simulink model "GCI_Ctrl_PLL_C2000"  (R2024a)
settings: Solver=FixedStepDiscrete  StartTime=0.0  StopTime=8  FixedStep=Sim.ContSampleTime  RelTol=1e-3  EnableMultiTasking=on
values from neighbouring files (symbols this model uses):
  ADPTV = 1.3912    [ModelDD.sldd]
  Ctrl = 0    [ModelDD.sldd]
  EnableMonitors = 0    [ModelDD.sldd]
  FrcPwr = 1    [ModelDD.sldd]
  IdSp = 0.0    [ModelDD.sldd]
  IqSp = 0.0    [ModelDD.sldd]
  ModReq = 1    [ModelDD.sldd]
  PorISel = 0    [ModelDD.sldd]
  PSp = 0.0    [ModelDD.sldd]
  QSp = 0.0    [ModelDD.sldd]
  Sim : value not decoded    [ModelDD.sldd]
  Test = 0    [ModelDD.sldd]
  Var = 650.0    [ModelDD.sldd]
undefined symbols (not defined in the file or in its folder): DiscIntNeverNeededParam, Down, GPTRIP1SEL, GPTRIP2SEL, magnitude, P, TZ1, TZ2, Up
libraries: simulink x38, c2837xDlib x22, c2802xlib x15, slpidlib x9, spsMeanLib x9, spsCurrentMeasurementLib x7, spsThreePhaseVIMeasurementLib x5, spsVoltageMeasurementLib x5, spsTHDLib x4, spsSeriesRLCBranchLib x4, svdutilitieslib x3, c280xlib x3
(part 3 of 11)

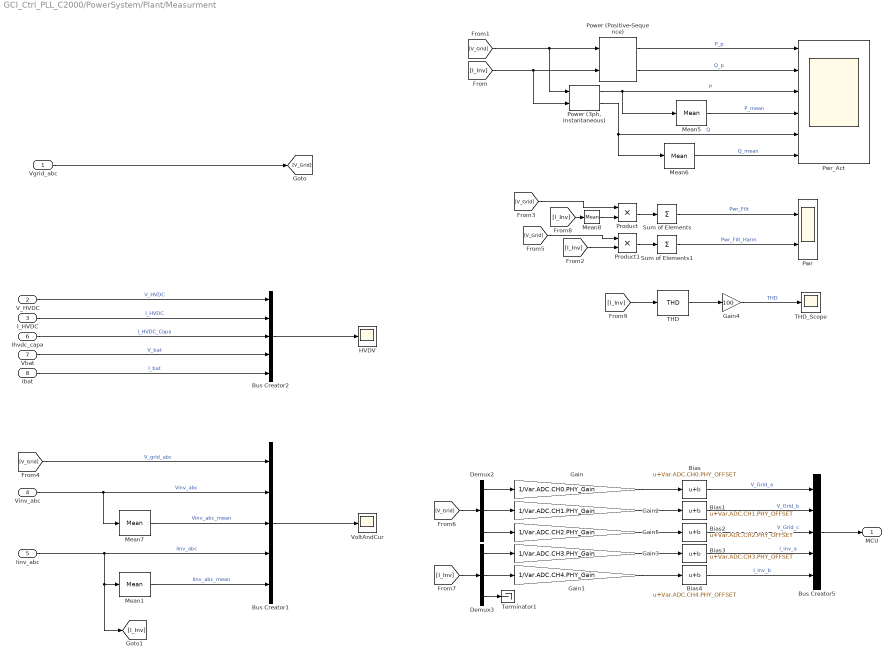
== system GCI_Ctrl_PLL_C2000/PowerSystem/Plant/Measurment ==
  Vgrid_abc : Inport
  V_HVDC : Inport  Port=2
  I_HVDC : Inport  Port=3
  Vinv_abc : Inport  Port=4
  Iinv_abc : Inport  Port=5
  Ihvdc_capa : Inport  Port=6
  Vbat : Inport  Port=7
  Ibat : Inport  Port=8
  Bias : Bias  Bias=Var.ADC.CH0.PHY_OFFSET  SaturateOnIntegerOverflow=off
  Bias1 : Bias  Bias=Var.ADC.CH1.PHY_OFFSET  SaturateOnIntegerOverflow=off
  Bias2 : Bias  Bias=Var.ADC.CH2.PHY_OFFSET  SaturateOnIntegerOverflow=off
  Bias3 : Bias  Bias=Var.ADC.CH3.PHY_OFFSET  SaturateOnIntegerOverflow=off
  Bias4 : Bias  Bias=Var.ADC.CH4.PHY_OFFSET  SaturateOnIntegerOverflow=off
  Bus Creator1 : BusCreator  Inputs=5
  Bus Creator2 : BusCreator  Inputs=5
  Bus Creator5 : BusCreator  Inputs=5
  Demux2 : Demux  Outputs=3
  Demux3 : Demux  Outputs=3
  Gain : Gain  Gain=1/Var.ADC.CH0.PHY_Gain
  Gain1 : Gain  Gain=1/Var.ADC.CH4.PHY_Gain
  Gain2 : Gain  Gain=1/Var.ADC.CH1.PHY_Gain
  Gain3 : Gain  Gain=1/Var.ADC.CH3.PHY_Gain
  Gain4 : Gain  Gain=100
  Gain5 : Gain  Gain=1/Var.ADC.CH2.PHY_Gain
  HVDV : Scope
  Mean1 : spsMeanLib/Mean  Freq=double(Var.PWM.Freq)  Vinit=0  Ts=0
  Mean5 : spsMeanLib/Mean  Freq=double(Var.Grid.Frq )  Vinit=0  Ts=0
  Mean6 : spsMeanLib/Mean  Freq=double(Var.Grid.Frq )  Vinit=0  Ts=0
  Mean7 : spsMeanLib/Mean  Freq=double(Var.PWM.Freq)  Vinit=0  Ts=0
  Mean8 : spsMeanLib/Mean  Freq="double(Var.PWM.Freq  )"  Vinit=0  Ts=0
  "Power (3ph, Instantaneous)" : spsPower3phInstantaneousLib/Power (3ph, Instantaneous)
  Power (Positive-Sequence) : spsPowerPositiveSequenceLib/Power (Positive-Sequence)  Freq=double(Var.Grid.Frq )  Vinit=[0, 0]  Iinit=[0, 0]  Ts=0
      settings: LibrarySourceBlock=|
      | sps_lib/Sensors and Measurements/Power
      | (Positive-Sequence)
  Product : Product
  Product1 : Product
  Pwr : Scope  NumInputPorts=2
  Pwr_Act : Scope  NumInputPorts=6
  Sum of Elements : Sum  Inputs=+
  Sum of Elements1 : Sum  Inputs=+
  THD : spsTHDLib/THD  Freq=double(Var.Grid.Frq )  Ts=0
  THD_Scope : Scope
  Terminator1 : Terminator
  VoltAndCur : Scope
  MCU : Outport  VectorParamsAs1DForOutWhenUnconnected=off
  wires:
  Iinv_abc/1 -> [I_Inv], Mean1/1, Bus Creator1/4  "Iinv_abc"
  Mean1/1 -> Bus Creator1/5  "Iinv_abc_mean"
  Mean7/1 -> Bus Creator1/3  "Vinv_abc_mean"
  Vinv_abc/1 -> Mean7/1, Bus Creator1/2  "Vinv_abc"
  Bus Creator2/1 -> HVDV/1
  Bus Creator1/1 -> VoltAndCur/1
  V_HVDC/1 -> Bus Creator2/1  "V_HVDC"
  I_HVDC/1 -> Bus Creator2/2  "I_HVDC"
  [V_Grid] -> Demux2/1
  [I_Inv] -> Demux3/1
  Demux2/1 -> Gain/1
  Demux3/2 -> Gain1/1
  Gain1/1 -> Bias4/1
  Gain3/1 -> Bias3/1
  Bias1/1 -> Bus Creator5/2  "V_Grid_b"
  Bias/1 -> Bus Creator5/1  "V_Grid_a"
  Bus Creator5/1 -> MCU/1
  Ihvdc_capa/1 -> Bus Creator2/3  "I_HVDC_Capa"
  Vbat/1 -> Bus Creator2/4  "V_bat"
  Ibat/1 -> Bus Creator2/5  "I_bat"
  Gain/1 -> Bias/1
  Demux2/2 -> Gain2/1
  Demux2/3 -> Gain5/1
  Gain2/1 -> Bias1/1
  Demux3/3 -> Terminator1/1
  Demux3/1 -> Gain3/1
  Power (Positive-Sequence)/1 -> Pwr_Act/1  "P_p"
  Power (Positive-Sequence)/2 -> Pwr_Act/2  "Q_p"
  Product/1 -> Sum of Elements/1
  THD/1 -> Gain4/1
  Gain4/1 -> THD_Scope/1  "THD"
  [I_Inv] -> "Power (3ph, Instantaneous)"/2, Power (Positive-Sequence)/2
  [V_Grid] -> "Power (3ph, Instantaneous)"/1, Power (Positive-Sequence)/1
  "Power (3ph, Instantaneous)"/1 -> Mean5/1, Pwr_Act/3  "P"
  "Power (3ph, Instantaneous)"/2 -> Pwr_Act/5, Mean6/1  "Q"
  Mean5/1 -> Pwr_Act/4  "P_mean"
  Mean6/1 -> Pwr_Act/6  "Q_mean"
  Mean8/1 -> Product/2
  Product1/1 -> Sum of Elements1/1
  Sum of Elements/1 -> Pwr/1  "Pwr_Filt"
  Sum of Elements1/1 -> Pwr/2  "Pwr_Filt_Harm"
  [I_Inv] -> Product1/2
  [V_Grid] -> Product/1
  [V_Grid] -> Product1/1
  [I_Inv] -> Mean8/1
  [I_Inv] -> THD/1
  [V_Grid] -> Bus Creator1/1  "V_grid_abc"
  Vgrid_abc/1 -> [V_Grid]
  Gain5/1 -> Bias2/1
  Bias2/1 -> Bus Creator5/3  "V_Grid_c"
  Bias3/1 -> Bus Creator5/4  "I_inv_a"
  Bias4/1 -> Bus Creator5/5  "I_inv_b"

== system GCI_Ctrl_PLL_C2000/PowerSystem/Plant/PWMGen1 ==
  Duty : Inport
  Constant : Constant  Value=0.5
  Deadtime : Subsystem  Commented=on
  Gain1 : Gain  Gain=2
  GreaterThan : RelationalOperator  Operator=>  RndMeth=Simplest  InputSameDT=off
  Mux : Mux  Inputs=2
  NOT : Logic  Operator=NOT  IconShape=distinctive  AllPortsSameDT=off  OutDataTypeStr=boolean
  Repeating Sequence : simulink/Sources/Repeating Sequence  rep_seq_t=[0 0.5/5000 1/5000]  rep_seq_y=[0 100 0]
  Scope : Scope  NumInputPorts=3
  Selector : Selector  InputPortWidth=6  IndexOptions=Index vector (dialog)  Indices=[1 4 2 5 3 6]  OutputSizes=1
  Subtract : Sum  Inputs=+-
  PWM : Outport  VectorParamsAs1DForOutWhenUnconnected=off
  wires:
  Mux/1 -> Selector/1
  Selector/1 -> Subtract/1
  Duty/1 -> GreaterThan/1, Scope/1
  Subtract/1 -> Gain1/1
  NOT/1 -> Mux/2
  Constant/1 -> Subtract/2
  Repeating Sequence/1 -> GreaterThan/2, Scope/2
  Gain1/1 -> PWM/1, Scope/3
  GreaterThan/1 -> Mux/1, NOT/1

== system GCI_Ctrl_PLL_C2000/PowerSystem/Plant/PWMGen2 ==
  Duty : Inport
  Constant : Constant  Value=0.5
  Deadtime : Subsystem  Commented=on
  Gain1 : Gain  Gain=2
  GreaterThan : RelationalOperator  Operator=>  RndMeth=Simplest  InputSameDT=off
  GreaterThan1 : RelationalOperator  Operator=>  RndMeth=Simplest  InputSameDT=off
  Mux : Mux  Inputs=2
  Repeating Sequence : simulink/Sources/Repeating Sequence  rep_seq_t=[0 0.5/5000 1/5000]  rep_seq_y=[0 100 0]
  Scope : Scope  NumInputPorts=4
  Selector : Selector  InputPortWidth=6  IndexOptions=Index vector (dialog)  Indices=[1 4 2 5 3 6]  OutputSizes=1
  Selector1 : Selector  InputPortWidth=6  IndexOptions=Index vector (dialog)  Indices=[1 2 3]  OutputSizes=1
  Selector2 : Selector  InputPortWidth=6  IndexOptions=Index vector (dialog)  Indices=[4 5 6]  OutputSizes=1
  Subtract : Sum  Inputs=+-
  PWM : Outport  VectorParamsAs1DForOutWhenUnconnected=off
  wires:
  Mux/1 -> Selector/1
  Gain1/1 -> Scope/4, PWM/1
  Repeating Sequence/1 -> GreaterThan1/1, Scope/3, GreaterThan/2
  Constant/1 -> Subtract/2
  Subtract/1 -> Gain1/1
  Duty/1 -> Scope/1, Selector2/1, Selector1/1
  Selector1/1 -> Scope/2, GreaterThan/1
  Selector2/1 -> GreaterThan1/2
  GreaterThan/1 -> Mux/1
  GreaterThan1/1 -> Mux/2
  Selector/1 -> Subtract/1

== system GCI_Ctrl_PLL_C2000/C2000_SW/Control/CommunicationMode/Serial Receive ==
  SCI_Rx_INT : TriggerPort  TriggerType=function-call  VariantControl=Variant
  Byte Pack1 : svdutilitieslib/Byte Pack  maskPackedDataType=uint8  datatypes={'single'}  byteAlign=1  blockPlatform=tic2000
      settings: LibrarySourceBlock=c2000lib/Target Communication/Byte Pack
  Byte Pack2 : svdutilitieslib/Byte Pack  maskPackedDataType=uint8  datatypes={'uint16'}  byteAlign=1  blockPlatform=tic2000
      settings: LibrarySourceBlock=c2000lib/Target Communication/Byte Pack
  Byte Unpack1 : svdutilitieslib/Byte Unpack  dimensions={[4]}  datatypes={'single'}  byteAlign=4  blockPlatform=tic2000
      settings: LibrarySourceBlock=c2000lib/Target Communication/Byte Unpack
  Data Store Read : DataStoreRead  Commented=on  DataStoreName=QSp  IndexOptions=Index vector (dialog)  Indices=1  OutputSizes=1
  Data Store Read1 : DataStoreRead  Commented=on  DataStoreName=PSp  IndexOptions=Index vector (dialog)  Indices=1  OutputSizes=1
  Data Store Read10 : DataStoreRead  DataStoreName=Irms  IndexOptions=Index vector (dialog)  Indices=1  OutputSizes=1
  Data Store Read11 : DataStoreRead  DataStoreName=Vdc  IndexOptions=Index vector (dialog)  Indices=1  OutputSizes=1
  Data Store Read12 : DataStoreRead  DataStoreName=Vrms  IndexOptions=Index vector (dialog)  Indices=1  OutputSizes=1
  Data Store Read13 : DataStoreRead  DataStoreName=w  IndexOptions=Index vector (dialog)  Indices=1  OutputSizes=1
  Data Store Read14 : DataStoreRead  DataStoreName=FailSw  IndexOptions=Index vector (dialog)  Indices=1  OutputSizes=1
  Data Store Read15 : DataStoreRead  DataStoreName=FailHw  IndexOptions=Index vector (dialog)  Indices=1  OutputSizes=1
  Data Store Read16 : DataStoreRead  DataStoreName=Fail  IndexOptions=Index vector (dialog)  Indices=1  OutputSizes=1
  Data Store Read17 : DataStoreRead  DataStoreName=SafeSt  IndexOptions=Index vector (dialog)  Indices=1  OutputSizes=1
  Data Store Read18 : DataStoreRead  DataStoreName=CtrlEn  IndexOptions=Index vector (dialog)  Indices=1  OutputSizes=1
  Data Store Read19 : DataStoreRead  DataStoreName=PllEnFb  IndexOptions=Index vector (dialog)  Indices=1  OutputSizes=1
  Data Store Read2 : DataStoreRead  Commented=on  DataStoreName=IqSp  IndexOptions=Index vector (dialog)  Indices=1  OutputSizes=1
  Data Store Read20 : DataStoreRead  DataStoreName=Synch  IndexOptions=Index vector (dialog)  Indices=1  OutputSizes=1
  Data Store Read21 : DataStoreRead  DataStoreName=Mode  IndexOptions=Index vector (dialog)  Indices=1  OutputSizes=1
  Data Store Read3 : DataStoreRead  Commented=on  DataStoreName=IdSp  IndexOptions=Index vector (dialog)  Indices=1  OutputSizes=1
  Data Store Read4 : DataStoreRead  Commented=on  DataStoreName=FrcPwr  IndexOptions=Index vector (dialog)  Indices=1  OutputSizes=1
  Data Store Read5 : DataStoreRead  Commented=on  DataStoreName=TestTrig  IndexOptions=Index vector (dialog)  Indices=1  OutputSizes=1
  Data Store Read6 : DataStoreRead  Commented=on  DataStoreName=EnaMon  IndexOptions=Index vector (dialog)  Indices=1  OutputSizes=1
  Data Store Read7 : DataStoreRead  Commented=on  DataStoreName=EnaPLL  IndexOptions=Index vector (dialog)  Indices=1  OutputSizes=1
  Data Store Read8 : DataStoreRead  Commented=on  DataStoreName=Sel_P_I  IndexOptions=Index vector (dialog)  Indices=1  OutputSizes=1
  Data Store Read9 : DataStoreRead  Commented=on  DataStoreName=ModReq  IndexOptions=Index vector (dialog)  Indices=1  OutputSizes=1
  Data Store Write : DataStoreWrite  DataStoreName=FrcPwr  IndexOptions=Index vector (dialog)  Indices=1  OutputSizes=1
  Data Store Write1 : DataStoreWrite  DataStoreName=TestTrig  IndexOptions=Index vector (dialog)  Indices=1  OutputSizes=1
  Data Store Write12 : DataStoreWrite  DataStoreName=IdSp  IndexOptions=Index vector (dialog)  Indices=1  OutputSizes=1
  Data Store Write13 : DataStoreWrite  DataStoreName=IqSp  IndexOptions=Index vector (dialog)  Indices=1  OutputSizes=1
  Data Store Write14 : DataStoreWrite  DataStoreName=PSp  IndexOptions=Index vector (dialog)  Indices=1  OutputSizes=1
  Data Store Write15 : DataStoreWrite  DataStoreName=QSp  IndexOptions=Index vector (dialog)  Indices=1  OutputSizes=1
  Data Store Write2 : DataStoreWrite  DataStoreName=EnaPLL  IndexOptions=Index vector (dialog)  Indices=1  OutputSizes=1
  Data Store Write3 : DataStoreWrite  DataStoreName=EnaMon  IndexOptions=Index vector (dialog)  Indices=1  OutputSizes=1
  Data Store Write4 : DataStoreWrite  DataStoreName=ModReq  IndexOptions=Index vector (dialog)  Indices=1  OutputSizes=1
  Data Store Write5 : DataStoreWrite  DataStoreName=Sel_P_I  IndexOptions=Index vector (dialog)  Indices=1  OutputSizes=1
  Data Type Conversion : DataTypeConversion  Commented=on  OutDataTypeStr=uint8  SaturateOnIntegerOverflow=off  RndMeth=Floor
  Demux : Demux
  Gain : Gain  Gain=single(2.^(0:4))  ParamDataTypeStr=single
  Mux : Mux  Commented=on
  Mux1 : Mux  Commented=on  Inputs=6
  Mux2 : Mux  Inputs=2
  Mux3 : Mux
  Mux4 : Mux  Inputs=5
  Mux5 : Mux
  SCI Receive : c280xlib/SCI Receive  sciModule=A  dataHead='SS'  headerCheckMaxCount=16  dataTail='EE'  dataType=uint8  dataLenOptions=Length via dialog  dataDim=17  maxDataLength=1  initValue=0  errOption=Output the last received value  errValue=0  sampleTime=-1  blockingMode=on  timeOut=1  outputStatus=off
  SCI Transmit : c280xlib/SCI Transmit  sciModule=A  dataHead='SS'  dataTail='EE'  frameSize=1  blockingMode=on  outputStatus=off
  Selector : Selector  InputPortWidth=17  IndexOptions=Index vector (dialog)  Indices=1:16  OutputSizes=1
  Selector1 : Selector  InputPortWidth=17  IndexOptions=Index vector (dialog)  Indices=17  OutputSizes=1
  Sum of Elements : Sum  Inputs=+  OutDataTypeStr=uint8
  unParse : Subsystem
  wires:
  Selector1/1 -> unParse/1(Data)
  unParse/1(ForcePwr) -> Data Store Write/1
  unParse/5(P_or_I) -> Data Store Write5/1
  unParse/2(TestTrigger) -> Data Store Write1/1
  unParse/3(EnaMon) -> Data Store Write3/1
  unParse/4(EnaPLL) -> Data Store Write2/1
  SCI Receive/1 -> Selector1/1, Selector/1
  Byte Unpack1/1 -> Demux/1
  Demux/2 -> Data Store Write13/1
  Demux/1 -> Data Store Write12/1
  Demux/3 -> Data Store Write14/1
  Demux/4 -> Data Store Write15/1
  Data Store Read/1 -> Mux/4
  Data Store Read1/1 -> Mux/3
  Data Store Read2/1 -> Mux/2
  Data Store Read3/1 -> Mux/1
  Mux3/1 -> Byte Pack1/1
  Selector/1 -> Byte Unpack1/1
  Data Store Read4/1 -> Mux1/1
  Data Store Read5/1 -> Mux1/2
  Data Store Read6/1 -> Mux1/3
  Data Store Read7/1 -> Mux1/4
  Data Store Read8/1 -> Mux1/5
  Mux1/1 -> Data Type Conversion/1
  Mux5/1 -> Mux2/2
  unParse/6(Mod) -> Data Store Write4/1
  Data Store Read9/1 -> Mux1/6
  Byte Pack1/1 -> Mux2/1  "Transmitted signal"
  Mux2/1 -> SCI Transmit/1
  Data Store Read10/1 -> Mux3/1
  Data Store Read11/1 -> Mux3/2
  Data Store Read12/1 -> Mux3/3
  Data Store Read13/1 -> Mux3/4
  Gain/1 -> Sum of Elements/1
  Data Store Read16/1 -> Mux4/1
  Data Store Read17/1 -> Mux4/2
  Data Store Read20/1 -> Mux4/3
  Data Store Read18/1 -> Mux4/4
  Data Store Read19/1 -> Mux4/5
  Mux4/1 -> Gain/1
  Data Store Read14/1 -> Byte Pack2/1
  Data Store Read21/1 -> Mux5/1
  Sum of Elements/1 -> Mux5/4
  Data Store Read15/1 -> Mux5/3
  Byte Pack2/1 -> Mux5/2  "Transmitted signal"

== system GCI_Ctrl_PLL_C2000/C2000_SW/CtrlLoop/ADC Scaling/ADC Scaling 3 Cur ==
  note: Data Collection
  note: Data Collection
  Ch1 : Inport
  Ch2 : Inport  Port=2
  Ch3 : Inport  Port=3
  Ch4 : Inport  Port=4
  Ch5 : Inport  Port=5
  Ch6 : Inport  Port=6
  SPO : Inport  Port=7
  PllEn : Inport  Port=8
  Add5 : Sum  Inputs=--  OutDataTypeStr=single
  Bus Creator : BusCreator  Commented=on  Inputs=6
  Bus Creator1 : BusCreator  Inputs=8
  Bus Selector : BusSelector  OutputSignals=VaActMeas
  Bus Selector1 : BusSelector  OutputSignals=VbActMeas
  Bus Selector2 : BusSelector  OutputSignals=IaActMeas
  Bus Selector3 : BusSelector  OutputSignals=IbActMeas
  Bus Selector4 : BusSelector  OutputSignals=IcActMeas
  Bus Selector5 : BusSelector  OutputSignals=VdcActMeas
  From : From  Commented=on  GotoTag=VaMeas
  From1 : From  Commented=on  GotoTag=VbMeas
  From2 : From  Commented=on  GotoTag=VcMeas
  From3 : From  Commented=on  GotoTag=IaMeas
  From4 : From  Commented=on  GotoTag=IbMeas
  From5 : From  Commented=on  GotoTag=VdcMeas
  Mux : Mux  Inputs=3
  Mux1 : Mux  Inputs=3
  NOT : Logic  Commented=on  Operator=NOT  IconShape=distinctive  AllPortsSameDT=off  OutDataTypeStr=boolean
  RemoveDCOffset : Subsystem  Variant=on  VariantControl=Variant1
      settings: PortSchema="{\"entries\":[{\"content\":{\"sides\":[{\"content\":{\"connectorIds\":[\"In1\"]},\"type\":\"ConnectorPlacement.EquallySpacedRectSide\",\"uuid\":\"cc4d9f7f-47aa-49df-af9b-f6b1a27a89d1\"},{\"content\":{\"connectorIds\":[\"Out1\",\"Out2\"],\"side\":\"RIGHT\"},\"type\":\"ConnectorPlacement.EquallySpacedRectSide\",\"uuid\":\"3802b5cc-b213-4712-8426-72153f4334cb\"},{\"content\":{\"connectorIds\":[\"In2\"],\"side\":\"TOP\"},\"type\":\"ConnectorPlacement.EquallySpacedRectSide\",\"uuid\":\"ab2b61dd-4b54-4d07-8aa7-d75851ccd714\"}]},\"type\":\"ConnectorPlacement.EquallySpacedConnector\",\"uuid\":\"275358d2-d3f0-4fc6-bdde-8d29d39068fc\"}],\"packageUris\":[\"http://schema.mathworks.com/mf0/Connector/R2020b\"],\"version\":\"1.0\"}"
  Scaling : Subsystem  mask{ADC_Gain=Var.ADC_CH0_Gain, ADC_Off=Var.ADC_CH0_OFFSET, Res=Var.ADC_Res, ADC_Gain_Phy=Var.ADC_CH0_PHY_Gain, ADC_Off_Phy=Var.ADC_CH0_PHY_OFFSET}
      mask prompts: ADC_Gain "ADC Gain"; ADC_Off "ADC Offset"; Res "Resoloution"; ADC_Gain_Phy "Physical Gain"; ADC_Off_Phy "Physical Offset"
  Scaling1 : Subsystem  mask{ADC_Gain=Var.ADC_CH1_Gain, ADC_Off=Var.ADC_CH1_OFFSET, Res=Var.ADC_Res, ADC_Gain_Phy=Var.ADC_CH1_PHY_Gain, ADC_Off_Phy=Var.ADC_CH1_PHY_OFFSET}
      mask prompts: ADC_Gain "ADC Gain"; ADC_Off "ADC Offset"; Res "Resoloution"; ADC_Gain_Phy "Physical Gain"; ADC_Off_Phy "Physical Offset"
  Scaling2 : Subsystem  mask{ADC_Gain=Var.ADC_CH2_Gain, ADC_Off=Var.ADC_CH2_OFFSET, Res=Var.ADC_Res, ADC_Gain_Phy=Var.ADC_CH2_PHY_Gain, ADC_Off_Phy=Var.ADC_CH2_PHY_OFFSET}
      mask prompts: ADC_Gain "ADC Gain"; ADC_Off "ADC Offset"; Res "Resoloution"; ADC_Gain_Phy "Physical Gain"; ADC_Off_Phy "Physical Offset"
  Scaling3 : Subsystem  mask{ADC_Gain=Var.ADC_CH3_Gain, ADC_Off=Var.ADC_CH3_OFFSET, Res=Var.ADC_Res, ADC_Gain_Phy=Var.ADC_CH3_PHY_Gain, ADC_Off_Phy=Var.ADC_CH3_PHY_OFFSET}
      mask prompts: ADC_Gain "ADC Gain"; ADC_Off "ADC Offset"; Res "Resoloution"; ADC_Gain_Phy "Physical Gain"; ADC_Off_Phy "Physical Offset"
  Scaling4 : Subsystem  mask{ADC_Gain=Var.ADC_CH4_Gain, ADC_Off=Var.ADC_CH4_OFFSET, Res=Var.ADC_Res, ADC_Gain_Phy=Var.ADC_CH4_PHY_Gain, ADC_Off_Phy=Var.ADC_CH4_PHY_OFFSET}
      mask prompts: ADC_Gain "ADC Gain"; ADC_Off "ADC Offset"; Res "Resoloution"; ADC_Gain_Phy "Physical Gain"; ADC_Off_Phy "Physical Offset"
  Scaling5 : Subsystem  mask{ADC_Gain=Var.ADC_CH5_Gain, ADC_Off=Var.ADC_CH5_OFFSET, Res=Var.ADC_Res, ADC_Gain_Phy=Var.ADC_CH5_PHY_Gain, ADC_Off_Phy=Var.ADC_CH5_PHY_OFFSET}
      mask prompts: ADC_Gain "ADC Gain"; ADC_Off "ADC Offset"; Res "Resoloution"; ADC_Gain_Phy "Physical Gain"; ADC_Off_Phy "Physical Offset"
  Subsystem : Subsystem
  Sum : Sum  Inputs=|+-
  Terminator : Terminator
  Unit Delay : UnitDelay  Commented=on  SampleTime=-1  HasFrameUpgradeWarning=on
  Vgrid_abc : Outport  OutDataTypeStr=single  VectorParamsAs1DForOutWhenUnconnected=off
  I_abc : Outport  Port=2  OutDataTypeStr=single  VectorParamsAs1DForOutWhenUnconnected=off
  Vhvdc : Outport  Port=3  OutDataTypeStr=single  VectorParamsAs1DForOutWhenUnconnected=off
  Mon : Outport  Port=4  OutDataTypeStr=single  VectorParamsAs1DForOutWhenUnconnected=off
  wires:
  RemoveDCOffset/2(VabcGridOff) -> Terminator/1
  NOT/1 -> Unit Delay/1
  Unit Delay/1 -> NOT/1
  SPO/1 -> Subsystem/Enable
  Subsystem/1(Offset) -> Sum/2
  Sum/1 -> I_abc/1, Bus Creator1/8  "Iabc_NoDcOff"
  RemoveDCOffset/1(VabcGridAdj) -> Bus Creator1/7, Vgrid_abc/1  "Vabc_NoDcOff"
  Bus Selector5/1 -> Bus Creator1/6  "<VdcActMeas>"
  Bus Selector4/1 -> Bus Creator1/5  "<IcActMeas>"
  Bus Selector3/1 -> Bus Creator1/4  "<IbActMeas>"
  Bus Selector2/1 -> Bus Creator1/3  "<IaActMeas>"
  Bus Selector1/1 -> Bus Creator1/2  "<VbActMeas>"
  Bus Selector/1 -> Bus Creator1/1  "<VaActMeas>"
  [VbMeas] -> Bus Selector1/1
  [VaMeas] -> Bus Selector/1
  [IaMeas] -> Bus Selector2/1
  [IcMeas] -> Bus Selector4/1
  [VdcMeas] -> Bus Selector5/1
  [IbMeas] -> Bus Selector3/1
  Ch4/1 -> Scaling3/1(CH)
  From5/1 -> Bus Creator/6
  Scaling5/2(CH_Meas) -> Vhvdc/1
  Scaling5/1(Meas) -> [VdcMeas]
  Ch6/1 -> Scaling5/1(CH)
  From3/1 -> Bus Creator/4
  From2/1 -> Bus Creator/3
  From4/1 -> Bus Creator/5
  From/1 -> Bus Creator/1
  Scaling4/2(CH_Meas) -> Mux1/3
  Scaling1/2(CH_Meas) -> Mux/2, Add5/2
  Scaling2/1(Mon) -> [IaMeas]
  Scaling3/2(CH_Meas) -> Mux1/2
  Ch5/1 -> Scaling4/1(CH)
  Scaling4/1(Meas) -> [IcMeas]
  Scaling3/1(Meas) -> [IbMeas]
  Scaling1/1(Mon) -> [VbMeas]
  Scaling/2(CH_Meas) -> Add5/1, Mux/1
  Scaling/1(Mon) -> [VaMeas]
  Scaling2/2(CH_Meas) -> Mux1/1
  Mux1/1 -> Sum/1, Subsystem/1(IabcActMeas)  "IabcActMeas"
  Mux/1 -> RemoveDCOffset/1(VabcGrid)  "VgabcActMeas"
  Ch1/1 -> Scaling/1(CH)
  Ch3/1 -> Scaling2/1(CH)
  Ch2/1 -> Scaling1/1(CH)
  From1/1 -> Bus Creator/2
  Bus Creator1/1 -> Mon/1  "ScaleMon"
  Add5/1 -> Mux/3  "Vc"
  PllEn/1 -> [A1]
  [A1] -> RemoveDCOffset/2(Rst)

== system GCI_Ctrl_PLL_C2000/C2000_SW/CtrlLoop/ADC Scaling/ADC Scaling 3 Volts ==
  note: Data Collection
  note: Data Collection
  Ch1 : Inport
  Ch2 : Inport  Port=2
  Ch3 : Inport  Port=3
  Ch4 : Inport  Port=4
  Ch5 : Inport  Port=5
  Ch6 : Inport  Port=6
  SPO : Inport  Port=7
  Add5 : Sum  Inputs=--  OutDataTypeStr=single
  Bus Creator : BusCreator  Commented=on  Inputs=6
  Bus Creator1 : BusCreator  Inputs=8
  Bus Selector : BusSelector  OutputSignals=VaActMeas
  Bus Selector1 : BusSelector  OutputSignals=VbActMeas
  Bus Selector2 : BusSelector  OutputSignals=VcActMeas
  Bus Selector3 : BusSelector  OutputSignals=IaActMeas
  Bus Selector4 : BusSelector  OutputSignals=IbActMeas
  Bus Selector5 : BusSelector  OutputSignals=VdcActMeas
  From : From  Commented=on  GotoTag=VaMeas
  From1 : From  Commented=on  GotoTag=VbMeas
  From2 : From  Commented=on  GotoTag=VcMeas
  From3 : From  Commented=on  GotoTag=IaMeas
  From4 : From  Commented=on  GotoTag=IbMeas
  From5 : From  Commented=on  GotoTag=VdcMeas
  Mux : Mux  Inputs=3
  Mux1 : Mux  Inputs=3
  NOT : Logic  Commented=on  Operator=NOT  IconShape=distinctive  AllPortsSameDT=off  OutDataTypeStr=boolean
  RemoveDCOffset : Subsystem  Variant=on  VariantControl=Variant1
  Scaling : Subsystem  mask{ADC_Gain=Var.ADC_CH0_Gain, ADC_Off=Var.ADC_CH0_OFFSET, Res=Var.ADC_Res, ADC_Gain_Phy=Var.ADC_CH0_PHY_Gain, ADC_Off_Phy=Var.ADC_CH0_PHY_OFFSET}
      mask prompts: ADC_Gain "ADC Gain"; ADC_Off "ADC Offset"; Res "Resoloution"; ADC_Gain_Phy "Physical Gain"; ADC_Off_Phy "Physical Offset"
  Scaling1 : Subsystem  mask{ADC_Gain=Var.ADC_CH1_Gain, ADC_Off=Var.ADC_CH1_OFFSET, Res=Var.ADC_Res, ADC_Gain_Phy=Var.ADC_CH1_PHY_Gain, ADC_Off_Phy=Var.ADC_CH1_PHY_OFFSET}
      mask prompts: ADC_Gain "ADC Gain"; ADC_Off "ADC Offset"; Res "Resoloution"; ADC_Gain_Phy "Physical Gain"; ADC_Off_Phy "Physical Offset"
  Scaling2 : Subsystem  mask{ADC_Gain=Var.ADC_CH2_Gain, ADC_Off=Var.ADC_CH2_OFFSET, Res=Var.ADC_Res, ADC_Gain_Phy=Var.ADC_CH2_PHY_Gain, ADC_Off_Phy=Var.ADC_CH2_PHY_OFFSET}
      mask prompts: ADC_Gain "ADC Gain"; ADC_Off "ADC Offset"; Res "Resoloution"; ADC_Gain_Phy "Physical Gain"; ADC_Off_Phy "Physical Offset"
  Scaling3 : Subsystem  mask{ADC_Gain=Var.ADC_CH3_Gain, ADC_Off=Var.ADC_CH3_OFFSET, Res=Var.ADC_Res, ADC_Gain_Phy=Var.ADC_CH3_PHY_Gain, ADC_Off_Phy=Var.ADC_CH3_PHY_OFFSET}
      mask prompts: ADC_Gain "ADC Gain"; ADC_Off "ADC Offset"; Res "Resoloution"; ADC_Gain_Phy "Physical Gain"; ADC_Off_Phy "Physical Offset"
  Scaling4 : Subsystem  mask{ADC_Gain=Var.ADC_CH4_Gain, ADC_Off=Var.ADC_CH4_OFFSET, Res=Var.ADC_Res, ADC_Gain_Phy=Var.ADC_CH4_PHY_Gain, ADC_Off_Phy=Var.ADC_CH4_PHY_OFFSET}
      mask prompts: ADC_Gain "ADC Gain"; ADC_Off "ADC Offset"; Res "Resoloution"; ADC_Gain_Phy "Physical Gain"; ADC_Off_Phy "Physical Offset"
  Scaling5 : Subsystem  mask{ADC_Gain=Var.ADC_CH5_Gain, ADC_Off=Var.ADC_CH5_OFFSET, Res=Var.ADC_Res, ADC_Gain_Phy=Var.ADC_CH5_PHY_Gain, ADC_Off_Phy=Var.ADC_CH5_PHY_OFFSET}
      mask prompts: ADC_Gain "ADC Gain"; ADC_Off "ADC Offset"; Res "Resoloution"; ADC_Gain_Phy "Physical Gain"; ADC_Off_Phy "Physical Offset"
  Subsystem : Subsystem
  Sum : Sum  Inputs=|+-
  Terminator : Terminator
  Unit Delay : UnitDelay  Commented=on  SampleTime=-1  HasFrameUpgradeWarning=on
  Vgrid_abc : Outport  OutDataTypeStr=single  VectorParamsAs1DForOutWhenUnconnected=off
  I_abc : Outport  Port=2  OutDataTypeStr=single  VectorParamsAs1DForOutWhenUnconnected=off
  Vhvdc : Outport  Port=3  OutDataTypeStr=single  VectorParamsAs1DForOutWhenUnconnected=off
  Mon : Outport  Port=4  OutDataTypeStr=single  VectorParamsAs1DForOutWhenUnconnected=off
  wires:
  Bus Creator1/1 -> Mon/1  "ScaleMon"
  From1/1 -> Bus Creator/2
  Ch2/1 -> Scaling1/1(CH)
  Ch3/1 -> Scaling2/1(CH)
  Ch1/1 -> Scaling/1(CH)
  Mux/1 -> RemoveDCOffset/1(VabcGrid)  "VgabcActMeas"
  Mux1/1 -> Subsystem/1(IabcActMeas), Sum/1  "IabcActMeas"
  Add5/1 -> Mux1/3  "Ic"
  Scaling2/2(CH_Meas) -> Mux/3
  Scaling/1(Mon) -> [VaMeas]
  Scaling/2(CH_Meas) -> Mux/1
  Scaling1/1(Mon) -> [VbMeas]
  Scaling3/1(Meas) -> [IaMeas]
  Scaling4/1(Meas) -> [IbMeas]
  Ch5/1 -> Scaling4/1(CH)
  Scaling3/2(CH_Meas) -> Add5/1, Mux1/1
  Scaling2/1(Mon) -> [VcMeas]
  Scaling1/2(CH_Meas) -> Mux/2
  Scaling4/2(CH_Meas) -> Add5/2, Mux1/2
  From/1 -> Bus Creator/1
  From4/1 -> Bus Creator/5
  From2/1 -> Bus Creator/3
  From3/1 -> Bus Creator/4
  Ch6/1 -> Scaling5/1(CH)
  Scaling5/1(Meas) -> [VdcMeas]
  Scaling5/2(CH_Meas) -> Vhvdc/1
  From5/1 -> Bus Creator/6
  Ch4/1 -> Scaling3/1(CH)
  [IbMeas] -> Bus Selector4/1
  [VdcMeas] -> Bus Selector5/1
  [VcMeas] -> Bus Selector2/1
  [IaMeas] -> Bus Selector3/1
  [VaMeas] -> Bus Selector/1
  [VbMeas] -> Bus Selector1/1
  Bus Selector/1 -> Bus Creator1/1  "<VaActMeas>"
  Bus Selector1/1 -> Bus Creator1/2  "<VbActMeas>"
  Bus Selector2/1 -> Bus Creator1/3  "<VcActMeas>"
  Bus Selector3/1 -> Bus Creator1/4  "<IaActMeas>"
  Bus Selector4/1 -> Bus Creator1/5  "<IbActMeas>"
  Bus Selector5/1 -> Bus Creator1/6  "<VdcActMeas>"
  RemoveDCOffset/1(VabcGridAdj) -> Vgrid_abc/1, Bus Creator1/7  "Vabc_NoDcOff"
  Sum/1 -> Bus Creator1/8, I_abc/1  "Iabc_NoDcOff"
  Subsystem/1(Offset) -> Sum/2
  SPO/1 -> Subsystem/Enable
  Unit Delay/1 -> NOT/1
  NOT/1 -> Unit Delay/1
  RemoveDCOffset/2(VabcGridOff) -> Terminator/1

== system GCI_Ctrl_PLL_C2000/C2000_SW/CtrlLoop/ADCs/HW ==
  note: Data Collection
  Meas : Inport
  ADC1 : c2802xlib/ADC  Commented=on  blkParamProc=C2000_Type4  ADCModule=C  samplingMode=Single sample mode  ADCResolution=12-bit (Single-ended input)  useSOC1=SOC0  useSOC2=SOC0_SOC1  SOCAcquisitionWindow=75  SOCTriggerSource=ePWM4_ADCSOCA  SOCInterruptTrigger=No ADCINT  Ts=-1  dType=uint16  postInterrupt=off  interruptSel=ADCINT2  ADCINTContinuous=off  endma=off  chdma=1  conv1=ADCINA0  conv2=ADCINA0 and ADCINB0  conv1_Type4=ADCIN2  conv2_Type4=ADCIN2 and ADCIN3
  ADC10 : c2802xlib/ADC  blkParamProc=C2000_Type4  ADCModule=C  samplingMode=Single sample mode  ADCResolution=12-bit (Single-ended input)  useSOC1=SOC0  useSOC2=SOC0_SOC1  SOCAcquisitionWindow=75  SOCTriggerSource=ePWM4_ADCSOCA  SOCInterruptTrigger=No ADCINT  Ts=-1  dType=uint32  postInterrupt=off  interruptSel=ADCINT2  ADCINTContinuous=off  endma=off  chdma=1  conv1=ADCINA0  conv2=ADCINA0 and ADCINB0  conv1_Type4=ADCIN2  conv2_Type4=ADCIN2 and ADCIN3
  ADC11 : c2802xlib/ADC  blkParamProc=C2000_Type4  ADCModule=A  samplingMode=Single sample mode  ADCResolution=12-bit (Single-ended input)  useSOC1=SOC1  useSOC2=SOC0_SOC1  SOCAcquisitionWindow=75  SOCTriggerSource=ePWM4_ADCSOCA  SOCInterruptTrigger=No ADCINT  Ts=-1  dType=uint32  postInterrupt=off  interruptSel=ADCINT1  ADCINTContinuous=off  endma=off  chdma=1  conv1=ADCINA0  conv2=ADCINA0 and ADCINB0  conv1_Type4=ADCIN1  conv2_Type4=ADCIN4 and ADCIN5
  ADC12 : c2802xlib/ADC  blkParamProc=C2000_Type4  ADCModule=A  samplingMode=Single sample mode  ADCResolution=12-bit (Single-ended input)  useSOC1=SOC2  useSOC2=SOC0_SOC1  SOCAcquisitionWindow=75  SOCTriggerSource=ePWM4_ADCSOCA  SOCInterruptTrigger=No ADCINT  Ts=-1  dType=uint32  postInterrupt=off  interruptSel=ADCINT4  ADCINTContinuous=off  endma=off  chdma=1  conv1=ADCINA0  conv2=ADCINA0 and ADCINB0  conv1_Type4=ADCIN2  conv2_Type4=ADCIN4 and ADCIN5
  ADC2 : c2802xlib/ADC  Commented=on  blkParamProc=C2000_Type4  ADCModule=C  samplingMode=Single sample mode  ADCResolution=12-bit (Single-ended input)  useSOC1=SOC1  useSOC2=SOC0_SOC1  SOCAcquisitionWindow=75  SOCTriggerSource=ePWM4_ADCSOCA  SOCInterruptTrigger=No ADCINT  Ts=-1  dType=uint16  postInterrupt=off  interruptSel=ADCINT4  ADCINTContinuous=off  endma=off  chdma=1  conv1=ADCINA0  conv2=ADCINA0 and ADCINB0  conv1_Type4=ADCIN3  conv2_Type4=ADCIN4 and ADCIN5
  ADC3 : c2802xlib/ADC  blkParamProc=C2000_Type4  ADCModule=A  samplingMode=Single sample mode  ADCResolution=12-bit (Single-ended input)  useSOC1=SOC0  useSOC2=SOC0_SOC1  SOCAcquisitionWindow=75  SOCTriggerSource=ePWM4_ADCSOCA  SOCInterruptTrigger=No ADCINT  Ts=-1  dType=uint32  postInterrupt=off  interruptSel=ADCINT2  ADCINTContinuous=off  endma=off  chdma=1  conv1=ADCINA0  conv2=ADCINA0 and ADCINB0  conv1_Type4=ADCIN0  conv2_Type4=ADCIN2 and ADCIN3
  ADC4 : c2802xlib/ADC  Commented=on  blkParamProc=C2000_Type4  ADCModule=A  samplingMode=Single sample mode  ADCResolution=12-bit (Single-ended input)  useSOC1=SOC0  useSOC2=SOC0_SOC1  SOCAcquisitionWindow=75  SOCTriggerSource=ePWM4_ADCSOCA  SOCInterruptTrigger=No ADCINT  Ts=-1  dType=uint16  postInterrupt=off  interruptSel=ADCINT1  ADCINTContinuous=off  endma=off  chdma=1  conv1=ADCINA0  conv2=ADCINA0 and ADCINB0  conv1_Type4=ADCIN2  conv2_Type4=ADCIN2 and ADCIN3
  ADC5 : c2802xlib/ADC  blkParamProc=C2000_Type4  ADCModule=B  samplingMode=Single sample mode  ADCResolution=12-bit (Single-ended input)  useSOC1=SOC5  useSOC2=SOC0_SOC1  SOCAcquisitionWindow=75  SOCTriggerSource=ePWM4_ADCSOCA  SOCInterruptTrigger=No ADCINT  Ts=-1  dType=uint32  postInterrupt=off  interruptSel=ADCINT4  ADCINTContinuous=off  endma=off  chdma=1  conv1=ADCINA0  conv2=ADCINA0 and ADCINB0  conv1_Type4=ADCIN4  conv2_Type4=ADCIN4 and ADCIN5
  ADC6 : c2802xlib/ADC  Commented=on  blkParamProc=C2000_Type4  ADCModule=B  samplingMode=Single sample mode  ADCResolution=12-bit (Single-ended input)  useSOC1=SOC0  useSOC2=SOC0_SOC1  SOCAcquisitionWindow=75  SOCTriggerSource=ePWM4_ADCSOCA  SOCInterruptTrigger=No ADCINT  Ts=-1  dType=uint16  postInterrupt=off  interruptSel=ADCINT2  ADCINTContinuous=off  endma=off  chdma=1  conv1=ADCINA0  conv2=ADCINA0 and ADCINB0  conv1_Type4=ADCIN2  conv2_Type4=ADCIN2 and ADCIN3
  ADC7 : c2802xlib/ADC  Commented=on  blkParamProc=C2000_Type4  ADCModule=A  samplingMode=Single sample mode  ADCResolution=12-bit (Single-ended input)  useSOC1=SOC1  useSOC2=SOC0_SOC1  SOCAcquisitionWindow=75  SOCTriggerSource=ePWM4_ADCSOCA  SOCInterruptTrigger=No ADCINT  Ts=-1  dType=uint16  postInterrupt=off  interruptSel=ADCINT1  ADCINTContinuous=off  endma=off  chdma=1  conv1=ADCINA0  conv2=ADCINA0 and ADCINB0  conv1_Type4=ADCIN3  conv2_Type4=ADCIN4 and ADCIN5
  ADC8 : c2802xlib/ADC  Commented=on  blkParamProc=C2000_Type4  ADCModule=B  samplingMode=Single sample mode  ADCResolution=12-bit (Single-ended input)  useSOC1=SOC1  useSOC2=SOC0_SOC1  SOCAcquisitionWindow=75  SOCTriggerSource=ePWM4_ADCSOCA  SOCInterruptTrigger=No ADCINT  Ts=-1  dType=uint16  postInterrupt=off  interruptSel=ADCINT4  ADCINTContinuous=off  endma=off  chdma=1  conv1=ADCINA0  conv2=ADCINA0 and ADCINB0  conv1_Type4=ADCIN3  conv2_Type4=ADCIN4 and ADCIN5
  ADC9 : c2802xlib/ADC  blkParamProc=C2000_Type4  ADCModule=B  samplingMode=Single sample mode  ADCResolution=12-bit (Single-ended input)  useSOC1=SOC0  useSOC2=SOC0_SOC1  SOCAcquisitionWindow=75  SOCTriggerSource=ePWM4_ADCSOCA  SOCInterruptTrigger=No ADCINT  Ts=-1  dType=uint32  postInterrupt=off  interruptSel=ADCINT1  ADCINTContinuous=off  endma=off  chdma=1  conv1=ADCINA0  conv2=ADCINA0 and ADCINB0  conv1_Type4=ADCIN5  conv2_Type4=ADCIN2 and ADCIN3
  Goto : Goto  Commented=on  GotoTag=VaMeas
  Goto1 : Goto  Commented=on  GotoTag=VbMeas
  Goto2 : Goto  Commented=on  GotoTag=VcMeas
  Goto3 : Goto  Commented=on  GotoTag=IaMeas
  Goto4 : Goto  Commented=on  GotoTag=IbMeas
  Goto5 : Goto  Commented=on  GotoTag=VdcMeas
  Mux : Mux  Inputs=6
  Terminator : Terminator
  A_Ch2 : Outport  VectorParamsAs1DForOutWhenUnconnected=off
  B_Ch2 : Outport  Port=2  VectorParamsAs1DForOutWhenUnconnected=off
  C_Ch2 : Outport  Port=3  VectorParamsAs1DForOutWhenUnconnected=off
  A_Ch3 : Outport  Port=4  VectorParamsAs1DForOutWhenUnconnected=off
  B_Ch3 : Outport  Port=5  VectorParamsAs1DForOutWhenUnconnected=off
  C_Ch3 : Outport  Port=6  VectorParamsAs1DForOutWhenUnconnected=off
  ADCs : Outport  Port=7  VectorParamsAs1DForOutWhenUnconnected=off
  wires:
  ADC4/1 -> Goto/1  "AdcACh2Raw"
  ADC6/1 -> Goto1/1  "AdcBCh2Raw"
  ADC7/1 -> Goto3/1  "AdcACh3Raw"
  ADC8/1 -> Goto4/1  "AdcBCh3Raw"
  Meas/1 -> Terminator/1
  ADC1/1 -> Goto2/1  "AdcCCh2Raw"
  ADC2/1 -> Goto5/1  "AdcCCh3Raw"
  [VaMeas] -> Mux/1
  [VdcMeas] -> Mux/6
  [IaMeas] -> Mux/4
  [VbMeas] -> Mux/2
  [VcMeas] -> Mux/3
  [IbMeas] -> Mux/5
  Mux/1 -> ADCs/1  "MonAdcRaw"
  ADC5/1 -> C_Ch3/1, [VdcMeas]  "AdcCCh3Raw"
  ADC3/1 -> C_Ch2/1, [VcMeas]  "AdcCCh2Raw"
  ADC12/1 -> B_Ch3/1, [IbMeas]  "AdcBCh3Raw"
  ADC11/1 -> A_Ch3/1, [IaMeas]  "AdcACh3Raw"
  ADC10/1 -> B_Ch2/1, [VbMeas]  "AdcBCh2Raw"
  ADC9/1 -> A_Ch2/1, [VaMeas]  "AdcACh2Raw"

== system GCI_Ctrl_PLL_C2000/C2000_SW/CtrlLoop/ADCs/SIM ==
  note: Monitoring Data Collection
  Meas : Inport
  ADC_SIM : Subsystem  mask{ADC_Gain=Var.ADC_CH0_Gain, ADC_Off=Var.ADC_CH0_OFFSET, Res=Var.ADC_Res}
      mask prompts: ADC_Gain "ADC Gain"; ADC_Off "ADC Offset"; Res "Resoloution"
  ADC_SIM1 : Subsystem  mask{ADC_Gain=Var.ADC_CH1_Gain, ADC_Off=Var.ADC_CH1_OFFSET, Res=Var.ADC_Res}
      mask prompts: ADC_Gain "ADC Gain"; ADC_Off "ADC Offset"; Res "Resoloution"
  ADC_SIM2 : Subsystem  mask{ADC_Gain=Var.ADC_CH2_Gain, ADC_Off=Var.ADC_CH2_OFFSET, Res=Var.ADC_Res}
      mask prompts: ADC_Gain "ADC Gain"; ADC_Off "ADC Offset"; Res "Resoloution"
  ADC_SIM3 : Subsystem  mask{ADC_Gain=Var.ADC_CH3_Gain, ADC_Off=Var.ADC_CH3_OFFSET, Res=Var.ADC_Res}
      mask prompts: ADC_Gain "ADC Gain"; ADC_Off "ADC Offset"; Res "Resoloution"
  ADC_SIM4 : Subsystem  mask{ADC_Gain=Var.ADC_CH4_Gain, ADC_Off=Var.ADC_CH4_OFFSET, Res=Var.ADC_Res}
      mask prompts: ADC_Gain "ADC Gain"; ADC_Off "ADC Offset"; Res "Resoloution"
  ADC_SIM5 : Subsystem  mask{ADC_Gain=Var.ADC_CH5_Gain, ADC_Off=Var.ADC_CH5_OFFSET, Res=Var.ADC_Res}
      mask prompts: ADC_Gain "ADC Gain"; ADC_Off "ADC Offset"; Res "Resoloution"
  Bus Selector{,1..5} (6 alike) : BusSelector  OutputSignals=ADC
  Demux : Demux  Outputs=6
  Mux : Mux  Inputs=6
  A_Ch2 : Outport  VectorParamsAs1DForOutWhenUnconnected=off
  B_Ch2 : Outport  Port=2  VectorParamsAs1DForOutWhenUnconnected=off
  C_Ch2 : Outport  Port=3  VectorParamsAs1DForOutWhenUnconnected=off
  A_Ch3 : Outport  Port=4  VectorParamsAs1DForOutWhenUnconnected=off
  B_Ch3 : Outport  Port=5  VectorParamsAs1DForOutWhenUnconnected=off
  C_Ch3 : Outport  Port=6  VectorParamsAs1DForOutWhenUnconnected=off
  ADCs : Outport  Port=7  VectorParamsAs1DForOutWhenUnconnected=off
  wires:
  ADC_SIM1/2(CH_Meas) -> B_Ch2/1  "AdcBCh2Raw"
  Demux/2 -> ADC_SIM1/1(CH)  "SimSnsMeas_Vb"
  Demux/4 -> ADC_SIM2/1(CH)  "SimSnsMeas_Ia"
  Demux/5 -> ADC_SIM3/1(CH)  "SimSnsMeas_Ib"
  ADC_SIM3/2(CH_Meas) -> B_Ch3/1  "AdcBCh3Raw"
  Meas/1 -> Demux/1
  ADC_SIM1/1(Mon) -> [VbMeas]
  ADC_SIM/1(Mon) -> [VaMeas]
  ADC_SIM/2(CH_Meas) -> A_Ch2/1  "AdcACh2Raw"
  ADC_SIM2/2(CH_Meas) -> A_Ch3/1  "AdcACh3Raw"
  Demux/3 -> ADC_SIM4/1(CH)  "SimSnsMeas_Vc"
  ADC_SIM4/2(CH_Meas) -> C_Ch2/1  "AdcCCh2Raw"
  ADC_SIM2/1(Mon) -> [IaMeas]
  ADC_SIM3/1(Mon) -> [IbMeas]
  ADC_SIM4/1(Mon) -> [VcMeas]
  ADC_SIM5/1(Mon) -> [VdcMeas]
  ADC_SIM5/2(CH_Meas) -> C_Ch3/1  "AdcCCh3Raw"
  Demux/6 -> ADC_SIM5/1(CH)  "SimSnsMeas_Vdc"
  Demux/1 -> ADC_SIM/1(CH)  "SimSnsMeas_Va"
  [VdcMeas] -> Bus Selector5/1
  [VcMeas] -> Bus Selector2/1
  Mux/1 -> ADCs/1  "AdcMonRaw"
  [IbMeas] -> Bus Selector4/1
  [IaMeas] -> Bus Selector3/1
  [VbMeas] -> Bus Selector1/1
  [VaMeas] -> Bus Selector/1
  Bus Selector/1 -> Mux/1  "<ADC>"
  Bus Selector1/1 -> Mux/2  "<ADC>"
  Bus Selector2/1 -> Mux/3  "<ADC>"
  Bus Selector3/1 -> Mux/4  "<ADC>"
  Bus Selector4/1 -> Mux/5  "<ADC>"
  Bus Selector5/1 -> Mux/6  "<ADC>"

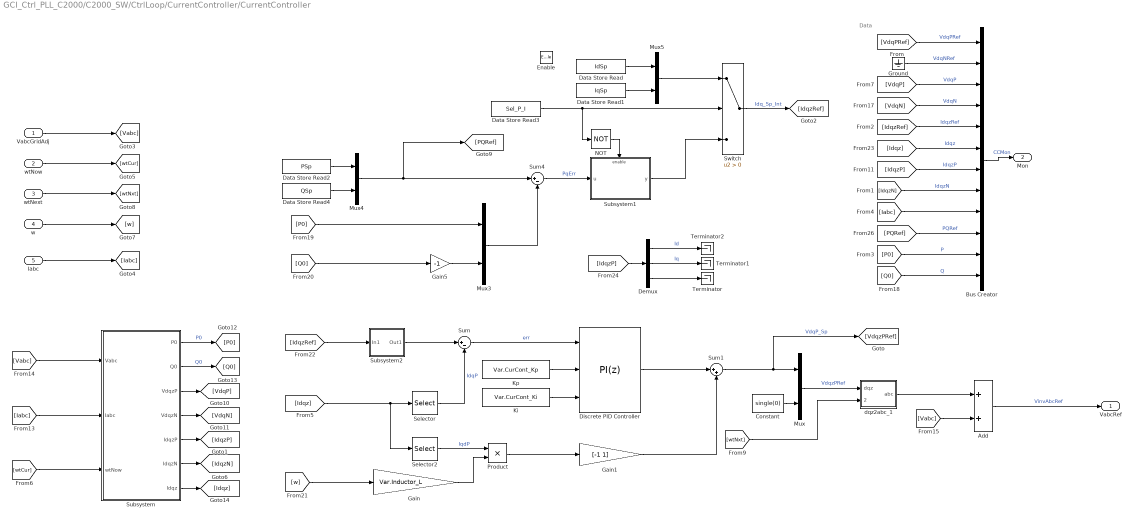
== system GCI_Ctrl_PLL_C2000/C2000_SW/CtrlLoop/CurrentController/CurrentController ==
  note: Data
  VabcGridAdj : Inport
  wtNow : Inport  Port=2
  wtNext : Inport  Port=3
  w : Inport  Port=4
  Iabc : Inport  Port=5
  Enable : EnablePort  StatesWhenEnabling=reset
  Add : Sum
  Bus Creator : BusCreator  Inputs=12
  Constant : Constant  Value=single(0)
  Data Store Read : DataStoreRead  DataStoreName=IdSp  IndexOptions=Index vector (dialog)  Indices=1  OutputSizes=1
  Data Store Read1 : DataStoreRead  DataStoreName=IqSp  IndexOptions=Index vector (dialog)  Indices=1  OutputSizes=1
  Data Store Read2 : DataStoreRead  DataStoreName=PSp  IndexOptions=Index vector (dialog)  Indices=1  OutputSizes=1
  Data Store Read3 : DataStoreRead  DataStoreName=Sel_P_I  IndexOptions=Index vector (dialog)  Indices=1  OutputSizes=1
  Data Store Read4 : DataStoreRead  DataStoreName=QSp  IndexOptions=Index vector (dialog)  Indices=1  OutputSizes=1
  Demux : Demux  Outputs=3
  Discrete PID Controller : slpidlib/PID Controller  Controller=PI  Form=Parallel  TimeDomain=Discrete-time  UseExternalTs=off  SampleTime=-1  IntegratorMethod=Forward Euler  FilterMethod=Forward Euler  ControllerParametersSource=external  P=1  I=1  UseKiTs=off  D=0  UseExternalDerivativeSource=off  N=100  UseFilter=on  TunerSelectOption=Transfer Function Based (PID Tuner App)  InitialConditionSource=internal  InitialConditionForIntegrator=0  InitialConditionForFilter=0  DifferentiatorICPrevScaledInput=0  ExternalReset=none  TrackingMode=off  Kt=1  LimitOutput=on  SatLimitsSource=internal  UpperSaturationLimit=Var.CurCont_MaxVdVq  LowerSaturationLimit=-Var.CurCont_MaxVdVq  LinearizeAsGain=on  AntiWindupMode=clamping  Kb=1  LimitIntegrator=off  UpperIntegratorSaturationLimit=inf  LowerIntegratorSaturationLimit=-inf  POutMin=[]  POutMax=[]  IOutMin=[]  IOutMax=[]  DOutMin=[]  DOutMax=[]  NOutMin=[]  NOutMax=[]  SumOutMin=[]  SumOutMax=[]  SaturationOutMin=[]  SaturationOutMax=[]  PParamMin=[]  PParamMax=[]  IParamMin=[]  IParamMax=[]  DParamMin=[]  DParamMax=[]  NParamMin=[]  NParamMax=[]  KbParamMin=[]  KbParamMax=[]  KtParamMin=[]  KtParamMax=[]  KbOutMin=[]  KbOutMax=[]  KtOutMin=[]  KtOutMax=[]  IntegratorOutMin=[]  IntegratorOutMax=[]  FilterOutMin=[]  FilterOutMax=[]  SumI1OutMin=[]  SumI1OutMax=[]  SumI2OutMin=[]  SumI2OutMax=[]  SumI3OutMin=[]  SumI3OutMax=[]  SumI4OutMin=[]  SumI4OutMax=[]  SumDOutMin=[]  SumDOutMax=[]  DifferentiatorOutMin=[]  DifferentiatorOutMax=[]  FilterDiffOutCoefMin=[]  FilterDiffOutCoefMax=[]  ReciprocalOutMin=[]  ReciprocalOutMax=[]  SumDenOutMin=[]  SumDenOutMax=[]  SumNumOutMin=[]  SumNumOutMax=[]  DivideOutMin=[]  DivideOutMax=[]  UdiffTsProdOutMin=[]  UdiffTsProdOutMax=[]  NTsProdOutMin=[]  NTsProdOutMax=[]  UintegralTsProdOutMin=[]  UintegralTsProdOutMax=[]  UngainTsProdOutMin=[]  UngainTsProdOutMax=[]  ClampingZeroOutDataTypeStr=Inherit: Inherit via back propagation  ClampingZeroOutMin=[]  ClampingZeroOutMax=[]  FilterDenConstantOutDataTypeStr=Inherit: Inherit via back propagation  FilterDenConstantOutMin=[]  FilterDenConstantOutMax=[]  PCopyOutDataTypeStr=Inherit: Inherit via back propagation  PCopyOutMin=[]  PCopyOutMax=[]  NCopyOutDataTypeStr=Inherit: Inherit via back propagation  NCopyOutMin=[]  NCopyOutMax=[]  IntegratorContinuousStateAttributes=''  IntegratorStateMustResolveToSignalObject=off  IntegratorRTWStateStorageClass=Auto  FilterContinuousStateAttributes=''  FilterStateMustResolveToSignalObject=off  FilterRTWStateStorageClass=Auto  ParallelPVariant=ExternalParameters  IdealPVariant=Disabled  IVariant=ExternalParameters  DVariant=Disabled  IntegratorVariant=Discrete  SatVariant=Enabled  AWVariant=DiscClampingParallel  PCopyVariant=Disabled  TRVariant=Disabled  FdbkBlocksVariant=Forward  IdealPFdbkVariant=Disabled  SatFdbkVariant=Disabled  DerivativeFilterVariant=Disabled  NVariant=Disabled  NCopyVariant=Disabled_SignalSpec  FilterICVariant=Disabled  IntegratorICVariant=InternalICs  ExternalResetVariant=Disabled  TRSumVariant=Passthrough  SumFdbkVariant=Disabled  SumVariant=Sum_PI  TsampFilterVariant=InternalTs  TsampNgainVariant=Passthrough  TsampIntegralVariant=Disabled_SignalSpec  ExternalSaturationOutDataTypeStr=Inherit: Same as second input  DerivativeSourceVariant=Disabled
  Gain : Gain  Gain=Var.Inductor_L
  Gain1 : Gain  Gain=[-1 1]  ParamDataTypeStr=single
  Gain5 : Gain  Gain=-1  ParamDataTypeStr=single
  Ground : Ground
  Ki : Constant  Value=Var.CurCont_Ki
  Kp : Constant  Value=Var.CurCont_Kp
  Mux{,3..5} (4 alike) : Mux  Inputs=2
  NOT : Logic  Operator=NOT  AllPortsSameDT=off  OutDataTypeStr=boolean
  Product : Product
  Selector : Selector  InputPortWidth=3  IndexOptions=Index vector (dialog)  Indices=[1 2]  OutputSizes=1
  Selector2 : Selector  InputPortWidth=3  IndexOptions=Index vector (dialog)  Indices=[2 1]  OutputSizes=1
  Subsystem : Subsystem
  Subsystem1 : Subsystem
  Subsystem2 : Subsystem
  Sum : Sum  Inputs=|+-
  Sum1 : Sum  Inputs=|++
  Sum4 : Sum  Inputs=|+-
  Switch : Switch  Criteria=u2 > Threshold  SaturateOnIntegerOverflow=off  InputSameDT=off
  Terminator : Terminator
  Terminator1 : Terminator
  Terminator2 : Terminator
  dqz2abc_1 : Subsystem
  VabcRef : Outport  VectorParamsAs1DForOutWhenUnconnected=off
  Mon : Outport  Port=2  VectorParamsAs1DForOutWhenUnconnected=off
  wires:
  [VdqP] -> Bus Creator/3  "VdqP"
  [wtNxt] -> dqz2abc_1/2(wtNext)
  VabcGridAdj/1 -> [Vabc]
  Sum4/1 -> Subsystem1/1(u)  "PqErr"
  [IdqzRef] -> Subsystem2/1(In1)
  Data Store Read3/1 -> NOT/1, Switch/2
  [Iabc] -> Subsystem/2(Iabc)
  [wtCur] -> Subsystem/3(wtNow)
  [Idqz] -> Selector/1, Selector2/1
  Subsystem1/1(y) -> Switch/3
  Ground/1 -> Bus Creator/2  "VdqNRef"
  Sum1/1 -> [VdqzPRef], Mux/1  "VdqP_Sp"
  Add/1 -> VabcRef/1  "VinvAbcRef"
  Iabc/1 -> [Iabc]
  [VdqN] -> Bus Creator/4  "VdqN"
  [Q0] -> Bus Creator/12  "Q"
  [P0] -> Bus Creator/11  "P"
  Switch/1 -> [IdqzRef]  "Idq_Sp_Int"
  [IdqzP] -> Bus Creator/7  "IdqzP"
  Gain/1 -> Product/2
  Mux/1 -> dqz2abc_1/1(dqz)  "VdqzPRef"
  Sum/1 -> Discrete PID Controller/1  "err"
  Mux3/1 -> Sum4/2
  dqz2abc_1/1(abc) -> Add/1
  [IdqzN] -> Bus Creator/8  "IdqzN"
  [Vabc] -> Add/2
  Demux/1 -> Terminator2/1  "Id"
  [Vabc] -> Subsystem/1(Vabc)
  Ki/1 -> Discrete PID Controller/3
  Product/1 -> Gain1/1
  Selector2/1 -> Product/1  "IqdP"
  Mux5/1 -> Switch/1
  [P0] -> Mux3/1
  [w] -> Gain/1
  [Q0] -> Gain5/1
  Kp/1 -> Discrete PID Controller/2
  Discrete PID Controller/1 -> Sum1/1
  Demux/3 -> Terminator/1
  Gain1/1 -> Sum1/2
  Subsystem/3(VdqzP) -> [VdqP]
  Subsystem/6(IdqzN) -> [IdqzN]
  wtNext/1 -> [wtNxt]
  [IdqzRef] -> Bus Creator/5  "IdqzRef"
  [VdqPRef] -> Bus Creator/1  "VdqPRef"
  w/1 -> [w]
  Demux/2 -> Terminator1/1  "Iq"
  Bus Creator/1 -> Mon/1  "CCMon"
  Subsystem/1(P0) -> [P0]  "P0"
  [Iabc] -> Bus Creator/9
  Constant/1 -> Mux/2
  Selector/1 -> Sum/2  "IdqP"
  Subsystem/5(IdqzP) -> [IdqzP]
  wtNow/1 -> [wtCur]
  Subsystem/4(VdqzN) -> [VdqN]
  Subsystem/2(Q0) -> [Q0]  "Q0"
  [Idqz] -> Bus Creator/6  "Idqz"
  Subsystem/7(Idqz) -> [Idqz]
  [IdqzP] -> Demux/1
  NOT/1 -> Subsystem1/Enable
  Gain5/1 -> Mux3/2
  Data Store Read1/1 -> Mux5/2
  Data Store Read/1 -> Mux5/1
  Data Store Read4/1 -> Mux4/2
  Data Store Read2/1 -> Mux4/1
  Subsystem2/1(Out1) -> Sum/1
  [PQRef] -> Bus Creator/10  "PQRef"
  Mux4/1 -> [PQRef], Sum4/1
